simulink model "AssembledTEST1"  (R2016b)
settings: Solver=VariableStepAuto  StartTime=0.0  StopTime=60  RelTol=1e-9
values from neighbouring files (symbols this model uses):
  DOWN_0 = -xtrim(12)    [Comparison_NonLin.m]    (also in InitialiseJ31.m = 1830.0192; Trim.m)
  EAST_0 = xtrim(11)    [Comparison_NonLin.m]    (also in InitialiseJ31.m = 0; Trim.m)
  FLAP = 0    [InitialiseJ31.m]
  INERTIA = [IXX,IXY,IXZ;IXY,IYY,IYZ;IXZ,IYZ,IZZ]    [InitialiseJ31.m]
  NORTH_0 = xtrim(10)    [Comparison_NonLin.m]    (also in InitialiseJ31.m = 0; Trim.m)
  P_0 = xtrim(4)    [Comparison_NonLin.m]    (also in InitialiseJ31.m = 0; Trim.m)
  PHI_0 = xtrim(7)    [Comparison_NonLin.m]    (also in Trim.m)
  PSI_0 = xtrim(9)    [Comparison_NonLin.m]    (also in Trim.m)
  Q_0 = xtrim(5)    [Comparison_NonLin.m]    (also in InitialiseJ31.m = 0; Trim.m)
  R2D = 180/pi    (= 57.2957795131)    [InitialiseJ31.m]
  R_0 = xtrim(6)    [Comparison_NonLin.m]    (also in InitialiseJ31.m = 0; Trim.m)
  THETA_0 = xtrim(8)    [Comparison_NonLin.m]    (also in Trim.m)
  U_0 = xtrim(1)    [Comparison_NonLin.m]    (also in Trim.m)
  V_0 = xtrim(2)    [Comparison_NonLin.m]    (also in Trim.m)
  W_0 = xtrim(3)    [Comparison_NonLin.m]    (also in Trim.m)
undefined symbols (not defined in the file or in its folder): ail_data, Ap, Aw, b, beta0_data, c0, c_i, cdrag_data, CG, clean_wing_data, crt, CT_data, D, D0q_10, D0q_20, D0q_35, DCDi_data, DCM0b, Deh_f_on_data, Deh_on_data, df, Dqhq_data, e0, e_data10, e_data20, e_data35, elaw_0, elaw_1, elaw_2, flaps_lift_data, flaps_moment_data, flaps_tail_data, flaps_wing_data, fmc_data, fmf_data, fmn_data, fus_data, gamma_t, h_data10, h_data20, h_data35, it, iw, Iwn2, J_W, K1_data, k1f_data, k_data, L_r0_10f, L_r0_20f, L_r0_35f, l_t, ld_data, Lt, Lt_dash, Lv_b, Lv_h, Lv_n, mac, mach_ffr ... (+39)
libraries: aerolibasang x3, aerolibatmos2 x1
(part 3 of 5)

== system AssembledTEST1/Subsystem/Longitudinal Aerodynamics/Get Wing XZM/Get XZM ==
  D : Inport
  L : Inport  Port=2
  alpha : Inport  Port=3
  M0 : Inport  Port=4
  x : Inport  Port=5
  z : Inport  Port=6
  Add : Sum  Inputs=--
  Add1 : Sum  Inputs=+-
  Add2 : Sum  Inputs=-++
  Product{,1..5} (6 alike) : Product  RndMeth=Zero
  Trigonometric Function : Trigonometry
  Trigonometric Function1 : Trigonometry  Operator=cos
  X : Outport
  Z : Outport  Port=2
  M : Outport  Port=3
  wires:
  alpha/1 -> Trigonometric Function/1, Trigonometric Function1/1
  L/1 -> Product1/1, Product/1
  Trigonometric Function1/1 -> Product/2, Product2/1
  Trigonometric Function/1 -> Product1/2, Product3/1
  D/1 -> Product3/2, Product2/2
  Add/1 -> Product4/1, Z/1
  Product/1 -> Add/1
  Product3/1 -> Add/2
  Product1/1 -> Add1/1
  Product2/1 -> Add1/2
  Add1/1 -> Product5/1, X/1
  Product4/1 -> Add2/1
  Product5/1 -> Add2/2
  x/1 -> Product4/2
  Add2/1 -> M/1
  z/1 -> Product5/2
  M0/1 -> Add2/3

== system AssembledTEST1/Subsystem/Longitudinal Aerodynamics/Get Wing XZM/get_M0w ==
  Mach : Inport
  Flap : Inport  Port=2
  qbar : Inport  Port=3
  Add : Sum
  Add1 : Sum
  Constant2 : Constant
  Constant3 : Constant  Value=0
  Constant5 : Constant  Value=Sw
  Constant6 : Constant  Value=mac
  Multiport Switch : MultiPortSwitch  Inputs=4
  Product : Product  Inputs=4  RndMeth=Zero
  get_CM0W : Lookup  InputValues=clean_wing_data(:,1)  Table=clean_wing_data(:,7)
  get_delCM0a10 : Lookup  InputValues=flaps_moment_data(:,1)  Table=flaps_moment_data(:,2)
  get_delCM0a20 : Lookup  InputValues=flaps_moment_data(:,1)  Table=flaps_moment_data(:,3)
  get_delCM0a35 : Lookup  InputValues=flaps_moment_data(:,1)  Table=flaps_moment_data(:,4)
  M0 : Outport
  wires:
  Mach/1 -> get_delCM0a35/1, get_delCM0a20/1, get_delCM0a10/1, get_CM0W/1
  Constant2/1 -> Add/1
  Add/1 -> Multiport Switch/1
  Constant3/1 -> Multiport Switch/2
  get_delCM0a10/1 -> Multiport Switch/3
  get_delCM0a20/1 -> Multiport Switch/4
  get_delCM0a35/1 -> Multiport Switch/5
  Add1/1 -> Product/1
  Constant5/1 -> Product/2
  Constant6/1 -> Product/4
  Product/1 -> M0/1
  qbar/1 -> Product/3
  Flap/1 -> Add/2
  Multiport Switch/1 -> Add1/2
  get_CM0W/1 -> Add1/1

== system AssembledTEST1/Subsystem/Longitudinal Aerodynamics/get_CDvwbasic/get_DelCL0tw ==
  flap : Inport
  Mach : Inport  Port=2
  Add : Sum
  Constant1 : Constant
  Constant6 : Constant  Value=0
  Multiport Switch1 : MultiPortSwitch  Inputs=4
  get_DelCL0_10 : Lookup  InputValues=flaps_lift_data(:,1)  Table=flaps_lift_data(:,8)
  get_DelCL0_20 : Lookup  InputValues=flaps_lift_data(:,1)  Table=flaps_lift_data(:,9)
  get_DelCL0_35 : Lookup  InputValues=flaps_lift_data(:,1)  Table=flaps_lift_data(:,10)
  DelCL0tw : Outport
  wires:
  Constant6/1 -> Multiport Switch1/2
  get_DelCL0_10/1 -> Multiport Switch1/3
  get_DelCL0_20/1 -> Multiport Switch1/4
  get_DelCL0_35/1 -> Multiport Switch1/5
  Mach/1 -> get_DelCL0_10/1, get_DelCL0_20/1, get_DelCL0_35/1
  Multiport Switch1/1 -> DelCL0tw/1
  Add/1 -> Multiport Switch1/1
  flap/1 -> Add/1
  Constant1/1 -> Add/2

== system AssembledTEST1/Subsystem/Longitudinal Aerodynamics/get_CDvwbasic/get_kf ==
  flap : Inport
  Mach : Inport  Port=2
  Add : Sum
  Constant1 : Constant
  Constant6 : Constant  Value=0
  Multiport Switch1 : MultiPortSwitch  Inputs=4
  get_DelCL0_35 : Lookup  InputValues=flaps_lift_data(:,1)  Table=flaps_lift_data(:,13)
  get_kf_10 : Lookup  InputValues=flaps_lift_data(:,1)  Table=flaps_lift_data(:,11)
  get_kf_20 : Lookup  InputValues=flaps_lift_data(:,1)  Table=flaps_lift_data(:,12)
  kf : Outport
  wires:
  Constant6/1 -> Multiport Switch1/2
  get_kf_10/1 -> Multiport Switch1/3
  get_kf_20/1 -> Multiport Switch1/4
  get_DelCL0_35/1 -> Multiport Switch1/5
  Mach/1 -> get_kf_10/1, get_kf_20/1, get_DelCL0_35/1
  Multiport Switch1/1 -> kf/1
  Add/1 -> Multiport Switch1/1
  flap/1 -> Add/1
  Constant1/1 -> Add/2

== system AssembledTEST1/Subsystem/Powerplants and Slipstream/Subsystem2/Get_delDi ==
  In2 : Inport
  In1 : Inport  Port=2
  In3 : Inport  Port=3
  In4 : Inport  Port=4
  In5 : Inport  Port=5
  In6 : Inport  Port=6
  In7 : Inport  Port=7
  In8 : Inport  Port=8
  Constant1 : Constant  Value=Aw
  Constant2 : Constant  Value=Sw
  Constant3 : Constant  Value=b
  Constant4 : Constant  Value=D
  Get KDi : Lookup  InputValues=DCDi_data(:,1)  Table=DCDi_data(:,2)
  Get bar e/ep : Lookup  InputValues=DCDi_data(:,1)  Table=DCDi_data(:,3)
  GetDelCDi : MATLAB Function  TreatAsAtomicUnit=on
  Out1 : Outport
  wires:
  In2/1 -> Get KDi/1, Get bar e/ep/1
  Get KDi/1 -> GetDelCDi/1(KDi)
  Get bar e/ep/1 -> GetDelCDi/3(bar_e_ep)
  Constant2/1 -> GetDelCDi/9(Sw)
  Constant1/1 -> GetDelCDi/10(Aw)
  Constant3/1 -> GetDelCDi/11(b)
  Constant4/1 -> GetDelCDi/13(D)
  In1/1 -> GetDelCDi/2(alpha)
  In3/1 -> GetDelCDi/4(Xp)
  In4/1 -> GetDelCDi/5(Zp)
  In5/1 -> GetDelCDi/6(CLw)
  In6/1 -> GetDelCDi/7(deu_dap)
  GetDelCDi/1(delDi) -> Out1/1
  In7/1 -> GetDelCDi/8(qbar)
  In8/1 -> GetDelCDi/12(CDiw)

== system AssembledTEST1/Subsystem/Powerplants and Slipstream/Subsystem2/Get_delDi1 ==
  In2 : Inport
  In1 : Inport  Port=2
  In3 : Inport  Port=3
  In4 : Inport  Port=4
  In5 : Inport  Port=5
  In6 : Inport  Port=6
  In7 : Inport  Port=7
  In8 : Inport  Port=8
  Constant1 : Constant  Value=Aw
  Constant2 : Constant  Value=Sw
  Constant3 : Constant  Value=b
  Constant4 : Constant  Value=D
  Get KDi : Lookup  InputValues=DCDi_data(:,1)  Table=DCDi_data(:,2)
  Get bar e/ep : Lookup  InputValues=DCDi_data(:,1)  Table=DCDi_data(:,3)
  GetDelCDi : MATLAB Function  TreatAsAtomicUnit=on
  Out1 : Outport
  wires:
  In2/1 -> Get KDi/1, Get bar e/ep/1
  Get KDi/1 -> GetDelCDi/1(KDi)
  Get bar e/ep/1 -> GetDelCDi/3(bar_e_ep)
  Constant2/1 -> GetDelCDi/9(Sw)
  Constant1/1 -> GetDelCDi/10(Aw)
  Constant3/1 -> GetDelCDi/11(b)
  Constant4/1 -> GetDelCDi/13(D)
  In1/1 -> GetDelCDi/2(alpha)
  In3/1 -> GetDelCDi/4(Xp)
  In4/1 -> GetDelCDi/5(Zp)
  In5/1 -> GetDelCDi/6(CLw)
  In6/1 -> GetDelCDi/7(deu_dap)
  GetDelCDi/1(delDi) -> Out1/1
  In7/1 -> GetDelCDi/8(qbar)
  In8/1 -> GetDelCDi/12(CDiw)

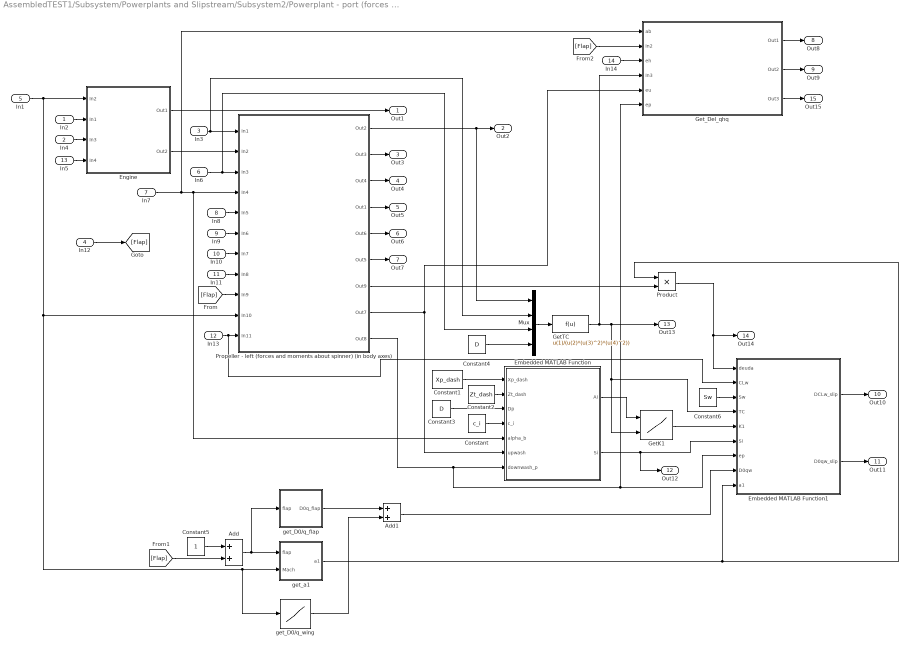
== system AssembledTEST1/Subsystem/Powerplants and Slipstream/Subsystem2/Powerplant - port (forces and moments about spinner) (in body axes) ==
  In2 : Inport
  In4 : Inport  Port=2
  In3 : Inport  Port=3
  In12 : Inport  Port=4
  In1 : Inport  Port=5
  In6 : Inport  Port=6
  In7 : Inport  Port=7
  In8 : Inport  Port=8
  In9 : Inport  Port=9
  In10 : Inport  Port=10
  In11 : Inport  Port=11
  In13 : Inport  Port=12
  In5 : Inport  Port=13
  In14 : Inport  Port=14
  Add : Sum
  Add1 : Sum
  Constant : Constant  Value=c_i
  Constant1 : Constant  Value=Xp_dash
  Constant2 : Constant  Value=Zt_dash
  Constant3 : Constant  Value=D
  Constant4 : Constant  Value=D
  Constant5 : Constant
  Constant6 : Constant  Value=Sw
  Embedded MATLAB Function : MATLAB Function  TreatAsAtomicUnit=on
  Embedded MATLAB Function1 : MATLAB Function  TreatAsAtomicUnit=on
  Engine : Subsystem
      mask Display:
      | port_label('output',1,'FFR [kg/h]')
      | port_label('output',2,'Power [SHP]')
      | port_label('input',1,'Mach')
      | port_label('input',2,'P_\infty [N/m^2]','texmode','on')
      | port_label('input',3,'T_\infty [K]','texmode','on')
      | port_label('input',4,'Throttle [%]')
  GetK1 : Lookup2D  RowIndex=Ai_ords  ColumnIndex=Tc_ords  Table=K1_data
  GetTC : Fcn  Expr=u(1)/(u(2)*(u(3)^2)*(u(4)^2))
  Get_Del_qhq : Subsystem
      mask Display:
      | port_label('output',1,'\Deltaq_h/q_\infty','texmode','on')
      | port_label('output',2,'(\Delta\epsilon_h)_{power}','texmode','on')
      | port_label('output',3,'\DeltaM_p/q_\infty','texmode','on')
      | port_label('input',1,'\alpha_b','texmode','on')
      | port_label('input',2,'Flap')
      | port_label('input',3,'(\epsilon_h)_{props off} [rad]','texmode','on')
      | port_label('input',4,'(S_W(T_c/prop))/(8R^2_p)','texmode','on')
      | port_label('input',5,'\epsilon_u [rad]','texmode','on')
      | port_label('input',6,'\epsilon_p [rad]','texmode','on')
  Mux : Mux
  Product : Product  RndMeth=Zero
  Propeller - left (forces and moments about spinner) (in body axes) : Subsystem
      mask Display:
      | port_label('output',1,'X [N]')
      | port_label('output',2,'Y [N]')
      | port_label('output',3,'Z [N]')
      | port_label('output',4,'L [Nm]')
      | port_label('output',5,'M [Nm]')
      | port_label('output',6,'N [Nm]')
      | port_label('output',8,'\epsilon_u [rad]','texmode','on')
      | port_label('output',9,'\epsilon_p [rad]','texmode','on')
      | port_label('output',7,'\delta\epsilon_u/\deltaC_L [rad]','texmode','on')
      | port_label('input',1,'\rho_\infty [kg/m^3]','texmode','on')
      | port_label('input',2,'Power [SHP]')
      | port_label('input',3,'V [m/s]')
      | port_label('input',4,'\alpha_b [rad]','texmode','on')
      | port_label('input',5,'\beta [rad]','texmode','on')
      | port_label('input',6,'p [rad/s]')
      | port_label('input',7,'q [rad/s]')
      | port_label('input',8,'r [rad/s]')
      | port_label('input',9,'Flap')
      | port_label('input',10,'Mach')
      | port_label('input',11,'C_{Lw}','texmode','on')
  get_D0/q_flap : Subsystem
  get_D0/q_wing : Lookup  InputValues=pdrag_data(:,1)  Table=pdrag_data(:,2)
  get_a1 : Subsystem
  Out1 : Outport
  Out2 : Outport  Port=2
  Out3 : Outport  Port=3
  Out4 : Outport  Port=4
  Out5 : Outport  Port=5
  Out6 : Outport  Port=6
  Out7 : Outport  Port=7
  Out8 : Outport  Port=8
  Out9 : Outport  Port=9
  Out10 : Outport  Port=10
  Out11 : Outport  Port=11
  Out12 : Outport  Port=12
  Out13 : Outport  Port=13
  Out14 : Outport  Port=14
  Out15 : Outport  Port=15
  wires:
  In1/1 -> Engine/1(In2), Propeller - left (forces and moments about spinner) (in body axes)/10(In10), get_a1/2(Mach), get_D0/q_wing/1
  Engine/2(Out2) -> Propeller - left (forces and moments about spinner) (in body axes)/2(In2)
  Engine/1(Out1) -> Out1/1
  In2/1 -> Engine/2(In1)
  In3/1 -> Propeller - left (forces and moments about spinner) (in body axes)/1(In1), Mux/2
  In4/1 -> Engine/3(In3)
  Propeller - left (forces and moments about spinner) (in body axes)/1(Out2) -> Out2/1, Mux/1
  In5/1 -> Engine/4(In4)
  In6/1 -> Propeller - left (forces and moments about spinner) (in body axes)/3(In3), Mux/3
  Propeller - left (forces and moments about spinner) (in body axes)/2(Out3) -> Out3/1
  In7/1 -> Propeller - left (forces and moments about spinner) (in body axes)/4(In4), Embedded MATLAB Function/5(alpha_b), Get_Del_qhq/1(ab)
  In8/1 -> Propeller - left (forces and moments about spinner) (in body axes)/5(In5)
  Propeller - left (forces and moments about spinner) (in body axes)/3(Out4) -> Out4/1
  In9/1 -> Propeller - left (forces and moments about spinner) (in body axes)/6(In6)
  In10/1 -> Propeller - left (forces and moments about spinner) (in body axes)/7(In7)
  Propeller - left (forces and moments about spinner) (in body axes)/4(Out1) -> Out5/1
  In11/1 -> Propeller - left (forces and moments about spinner) (in body axes)/8(In8)
  Propeller - left (forces and moments about spinner) (in body axes)/5(Out6) -> Out6/1
  Propeller - left (forces and moments about spinner) (in body axes)/6(Out5) -> Out7/1
  In13/1 -> Propeller - left (forces and moments about spinner) (in body axes)/11(In11), Embedded MATLAB Function1/2(CLw)
  Propeller - left (forces and moments about spinner) (in body axes)/8(Out7) -> Embedded MATLAB Function/6(upwash), Get_Del_qhq/5(eu)
  Propeller - left (forces and moments about spinner) (in body axes)/9(Out8) -> Embedded MATLAB Function/7(downwash_p), Get_Del_qhq/6(ep), Embedded MATLAB Function1/7(ep)
  Constant1/1 -> Embedded MATLAB Function/1(Xp_dash)
  Constant2/1 -> Embedded MATLAB Function/2(Zt_dash)
  Constant3/1 -> Embedded MATLAB Function/3(Dp)
  Constant/1 -> Embedded MATLAB Function/4(c_i)
  Embedded MATLAB Function/1(Ai) -> GetK1/1
  Mux/1 -> GetTC/1
  GetTC/1 -> GetK1/2, Embedded MATLAB Function1/4(TC), Out13/1, Get_Del_qhq/4(In3)
  Constant4/1 -> Mux/4
  Constant5/1 -> Add/1
  Add/1 -> get_a1/1(flap), get_D0/q_flap/1(flap)
  get_a1/1(a1) -> Product/1, Embedded MATLAB Function1/9(a1)
  Propeller - left (forces and moments about spinner) (in body axes)/7(Out9) -> Product/2
  Product/1 -> Out14/1, Embedded MATLAB Function1/1(deuda)
  Embedded MATLAB Function/2(Si) -> Out12/1, Embedded MATLAB Function1/6(Si)
  GetK1/1 -> Embedded MATLAB Function1/5(K1)
  Constant6/1 -> Embedded MATLAB Function1/3(Sw)
  get_D0/q_flap/1(D0q_flap) -> Add1/1
  get_D0/q_wing/1 -> Add1/2
  Add1/1 -> Embedded MATLAB Function1/8(D0qw)
  In12/1 -> [Flap]
  [Flap] -> Propeller - left (forces and moments about spinner) (in body axes)/9(In9)
  [Flap] -> Add/2
  [Flap] -> Get_Del_qhq/2(In2)
  In14/1 -> Get_Del_qhq/3(eh)
  Get_Del_qhq/1(Out1) -> Out8/1
  Embedded MATLAB Function1/1(DCLw_slip) -> Out10/1
  Embedded MATLAB Function1/2(D0qw_slip) -> Out11/1
  Get_Del_qhq/2(Out2) -> Out9/1
  Get_Del_qhq/3(Out3) -> Out15/1

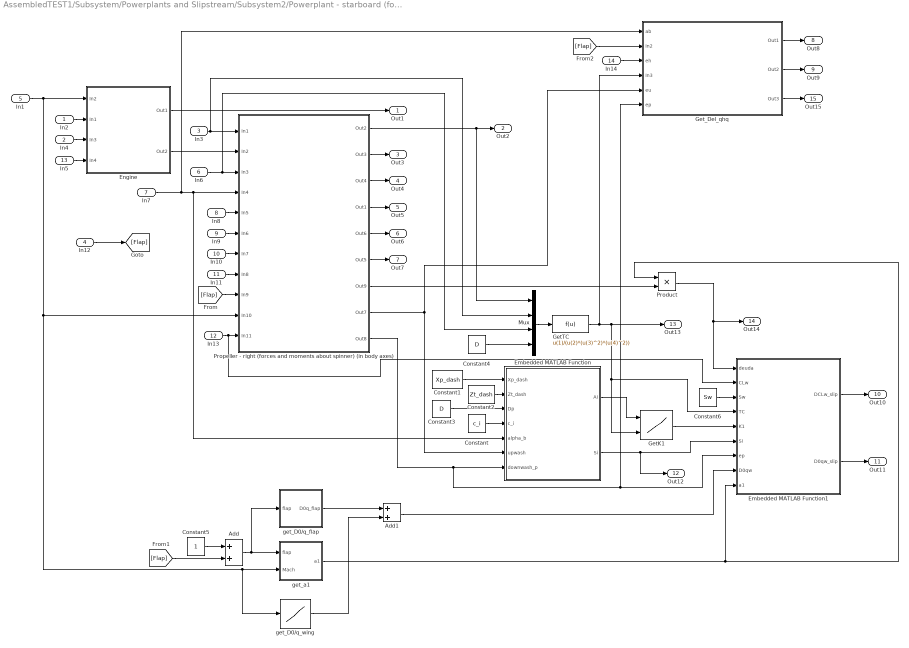
== system AssembledTEST1/Subsystem/Powerplants and Slipstream/Subsystem2/Powerplant - starboard (forces and moments about spinner) (in body axes) ==
  In2 : Inport
  In4 : Inport  Port=2
  In3 : Inport  Port=3
  In12 : Inport  Port=4
  In1 : Inport  Port=5
  In6 : Inport  Port=6
  In7 : Inport  Port=7
  In8 : Inport  Port=8
  In9 : Inport  Port=9
  In10 : Inport  Port=10
  In11 : Inport  Port=11
  In13 : Inport  Port=12
  In5 : Inport  Port=13
  In14 : Inport  Port=14
  Add : Sum
  Add1 : Sum
  Constant : Constant  Value=c_i
  Constant1 : Constant  Value=Xp_dash
  Constant2 : Constant  Value=Zt_dash
  Constant3 : Constant  Value=D
  Constant4 : Constant  Value=D
  Constant5 : Constant
  Constant6 : Constant  Value=Sw
  Embedded MATLAB Function : MATLAB Function  TreatAsAtomicUnit=on
  Embedded MATLAB Function1 : MATLAB Function  TreatAsAtomicUnit=on
  Engine : Subsystem
      mask Display:
      | port_label('output',1,'FFR [kg/h]')
      | port_label('output',2,'Power [SHP]')
      | port_label('input',1,'Mach')
      | port_label('input',2,'P_\infty [N/m^2]','texmode','on')
      | port_label('input',3,'T_\infty [K]','texmode','on')
      | port_label('input',4,'Throttle [%]')
  GetK1 : Lookup2D  RowIndex=Ai_ords  ColumnIndex=Tc_ords  Table=K1_data
  GetTC : Fcn  Expr=u(1)/(u(2)*(u(3)^2)*(u(4)^2))
  Get_Del_qhq : Subsystem
      mask Display:
      | port_label('output',1,'\Deltaq_h/q_\infty','texmode','on')
      | port_label('output',2,'(\Delta\epsilon_h)_{power}','texmode','on')
      | port_label('output',3,'\DeltaM_p/q_\infty','texmode','on')
      | port_label('input',1,'\alpha_b','texmode','on')
      | port_label('input',2,'Flap')
      | port_label('input',3,'(\epsilon_h)_{props off} [rad]','texmode','on')
      | port_label('input',4,'(S_W(T_c/prop))/(8R^2_p)','texmode','on')
      | port_label('input',5,'\epsilon_u [rad]','texmode','on')
      | port_label('input',6,'\epsilon_p [rad]','texmode','on')
  Mux : Mux
  Product : Product  RndMeth=Zero
  Propeller - right (forces and moments about spinner) (in body axes) : Subsystem
      mask Display:
      | port_label('output',1,'X [N]')
      | port_label('output',2,'Y [N]')
      | port_label('output',3,'Z [N]')
      | port_label('output',4,'L [Nm]')
      | port_label('output',5,'M [Nm]')
      | port_label('output',6,'N [Nm]')
      | port_label('output',8,'\epsilon_u [rad]','texmode','on')
      | port_label('output',9,'\epsilon_p [rad]','texmode','on')
      | port_label('output',7,'\delta\epsilon_u/\deltaC_L [rad]','texmode','on')
      | port_label('input',1,'\rho_\infty [kg/m^3]','texmode','on')
      | port_label('input',2,'Power [SHP]')
      | port_label('input',3,'V [m/s]')
      | port_label('input',4,'\alpha_b [rad]','texmode','on')
      | port_label('input',5,'\beta [rad]','texmode','on')
      | port_label('input',6,'p [rad/s]')
      | port_label('input',7,'q [rad/s]')
      | port_label('input',8,'r [rad/s]')
      | port_label('input',9,'Flap')
      | port_label('input',10,'Mach')
      | port_label('input',11,'C_{Lw}','texmode','on')
  get_D0/q_flap : Subsystem
  get_D0/q_wing : Lookup  InputValues=pdrag_data(:,1)  Table=pdrag_data(:,2)
  get_a1 : Subsystem
  Out1 : Outport
  Out2 : Outport  Port=2
  Out3 : Outport  Port=3
  Out4 : Outport  Port=4
  Out5 : Outport  Port=5
  Out6 : Outport  Port=6
  Out7 : Outport  Port=7
  Out8 : Outport  Port=8
  Out9 : Outport  Port=9
  Out10 : Outport  Port=10
  Out11 : Outport  Port=11
  Out12 : Outport  Port=12
  Out13 : Outport  Port=13
  Out14 : Outport  Port=14
  Out15 : Outport  Port=15
  wires:
  In1/1 -> Engine/1(In2), Propeller - right (forces and moments about spinner) (in body axes)/10(In10), get_a1/2(Mach), get_D0/q_wing/1
  Engine/2(Out2) -> Propeller - right (forces and moments about spinner) (in body axes)/2(In2)
  Engine/1(Out1) -> Out1/1
  In2/1 -> Engine/2(In1)
  In3/1 -> Propeller - right (forces and moments about spinner) (in body axes)/1(In1), Mux/2
  In4/1 -> Engine/3(In3)
  Propeller - right (forces and moments about spinner) (in body axes)/1(Out2) -> Out2/1, Mux/1
  In5/1 -> Engine/4(In4)
  In6/1 -> Propeller - right (forces and moments about spinner) (in body axes)/3(In3), Mux/3
  Propeller - right (forces and moments about spinner) (in body axes)/2(Out3) -> Out3/1
  In7/1 -> Propeller - right (forces and moments about spinner) (in body axes)/4(In4), Embedded MATLAB Function/5(alpha_b), Get_Del_qhq/1(ab)
  In8/1 -> Propeller - right (forces and moments about spinner) (in body axes)/5(In5)
  Propeller - right (forces and moments about spinner) (in body axes)/3(Out4) -> Out4/1
  In9/1 -> Propeller - right (forces and moments about spinner) (in body axes)/6(In6)
  In10/1 -> Propeller - right (forces and moments about spinner) (in body axes)/7(In7)
  Propeller - right (forces and moments about spinner) (in body axes)/4(Out1) -> Out5/1
  In11/1 -> Propeller - right (forces and moments about spinner) (in body axes)/8(In8)
  Propeller - right (forces and moments about spinner) (in body axes)/5(Out6) -> Out6/1
  Propeller - right (forces and moments about spinner) (in body axes)/6(Out5) -> Out7/1
  In13/1 -> Propeller - right (forces and moments about spinner) (in body axes)/11(In11), Embedded MATLAB Function1/2(CLw)
  Propeller - right (forces and moments about spinner) (in body axes)/8(Out7) -> Embedded MATLAB Function/6(upwash), Get_Del_qhq/5(eu)
  Propeller - right (forces and moments about spinner) (in body axes)/9(Out8) -> Embedded MATLAB Function/7(downwash_p), Get_Del_qhq/6(ep), Embedded MATLAB Function1/7(ep)
  Constant1/1 -> Embedded MATLAB Function/1(Xp_dash)
  Constant2/1 -> Embedded MATLAB Function/2(Zt_dash)
  Constant3/1 -> Embedded MATLAB Function/3(Dp)
  Constant/1 -> Embedded MATLAB Function/4(c_i)
  Embedded MATLAB Function/1(Ai) -> GetK1/1
  Mux/1 -> GetTC/1
  GetTC/1 -> Get_Del_qhq/4(In3), GetK1/2, Embedded MATLAB Function1/4(TC), Out13/1
  Constant4/1 -> Mux/4
  Constant5/1 -> Add/1
  Add/1 -> get_a1/1(flap), get_D0/q_flap/1(flap)
  get_a1/1(a1) -> Product/1, Embedded MATLAB Function1/9(a1)
  Propeller - right (forces and moments about spinner) (in body axes)/7(Out9) -> Product/2
  Product/1 -> Out14/1, Embedded MATLAB Function1/1(deuda)
  Embedded MATLAB Function/2(Si) -> Out12/1, Embedded MATLAB Function1/6(Si)
  GetK1/1 -> Embedded MATLAB Function1/5(K1)
  Constant6/1 -> Embedded MATLAB Function1/3(Sw)
  get_D0/q_flap/1(D0q_flap) -> Add1/1
  get_D0/q_wing/1 -> Add1/2
  Add1/1 -> Embedded MATLAB Function1/8(D0qw)
  In12/1 -> [Flap]
  [Flap] -> Propeller - right (forces and moments about spinner) (in body axes)/9(In9)
  [Flap] -> Add/2
  [Flap] -> Get_Del_qhq/2(In2)
  In14/1 -> Get_Del_qhq/3(eh)
  Get_Del_qhq/1(Out1) -> Out8/1
  Get_Del_qhq/2(Out2) -> Out9/1
  Embedded MATLAB Function1/1(DCLw_slip) -> Out10/1
  Embedded MATLAB Function1/2(D0qw_slip) -> Out11/1
  Get_Del_qhq/3(Out3) -> Out15/1

== system AssembledTEST1/Subsystem/Powerplants and Slipstream/Subsystem2/Subsystem ==
  In1 : Inport
  In2 : Inport  Port=2
  In5 : Inport  Port=3
  In3 : Inport  Port=4
  In4 : Inport  Port=5
  In6 : Inport  Port=6
  Add : Sum  Inputs=+-
  Add1 : Sum
  Constant : Constant
  Constant1 : Constant  Value=0.5
  Constant2 : Constant  Value=St
  Constant3 : Constant  Value=Sit
  Divide : Product  Inputs=*/***
  Product : Product  RndMeth=Zero
  Product1 : Product  RndMeth=Zero
  Product2 : Product  Inputs=4  RndMeth=Zero
  Out1 : Outport
  Out2 : Outport  Port=2
  wires:
  Product/1 -> Add/2
  Add/1 -> Product1/1
  Constant/1 -> Add1/2
  Add1/1 -> Product1/2
  Product1/1 -> Product2/1
  Constant1/1 -> Product2/2
  Constant2/1 -> Product2/3, Divide/2
  In1/1 -> Add/1
  In2/1 -> Product/1
  In3/1 -> Product/2
  Product2/1 -> Out1/1
  In4/1 -> Product2/4, Divide/1
  In5/1 -> Add1/1, Divide/4
  Divide/1 -> Out2/1
  Constant3/1 -> Divide/3
  In6/1 -> Divide/5

== system AssembledTEST1/Subsystem/Powerplants and Slipstream/Subsystem2/Subsystem1 ==
  In1 : Inport
  In2 : Inport  Port=2
  In5 : Inport  Port=3
  In3 : Inport  Port=4
  In4 : Inport  Port=5
  In6 : Inport  Port=6
  Add : Sum  Inputs=+-
  Add1 : Sum
  Constant : Constant
  Constant1 : Constant  Value=0.5
  Constant2 : Constant  Value=St
  Constant3 : Constant  Value=Sit
  Divide : Product  Inputs=*/***
  Product : Product  RndMeth=Zero
  Product1 : Product  RndMeth=Zero
  Product2 : Product  Inputs=4  RndMeth=Zero
  Out1 : Outport
  Out2 : Outport  Port=2
  wires:
  Product/1 -> Add/2
  Add/1 -> Product1/1
  Constant/1 -> Add1/2
  Add1/1 -> Product1/2
  Product1/1 -> Product2/1
  Constant1/1 -> Product2/2
  Constant2/1 -> Product2/3, Divide/2
  In1/1 -> Add/1
  In2/1 -> Product/1
  In3/1 -> Product/2
  Product2/1 -> Out1/1
  In4/1 -> Product2/4, Divide/1
  In5/1 -> Add1/1, Divide/4
  Divide/1 -> Out2/1
  Constant3/1 -> Divide/3
  In6/1 -> Divide/5

== system AssembledTEST1/Subsystem/Lateral//Directional Aerodynamics/getYLN/Subsystem/If Action Subsystem ==
  In1 : Inport
  Action Port : ActionPort  ActionType=else
  Out1 : Outport
  wires:
  In1/1 -> Out1/1

== system AssembledTEST1/Subsystem/Lateral//Directional Aerodynamics/getYLN/Subsystem/If Action Subsystem1 ==
  In1 : Inport
  Action Port : ActionPort  ActionType=then
  Out1 : Outport
  wires:
  In1/1 -> Out1/1

== system AssembledTEST1/Subsystem/Longitudinal Aerodynamics/Get Drag/get_CDvw/get_DelCL0tw ==
  flap : Inport
  Mach : Inport  Port=2
  Constant6 : Constant  Value=0
  Multiport Switch1 : MultiPortSwitch  Inputs=4
  get_DelCL0_10 : Lookup  InputValues=flaps_lift_data(:,1)  Table=flaps_lift_data(:,8)
  get_DelCL0_20 : Lookup  InputValues=flaps_lift_data(:,1)  Table=flaps_lift_data(:,9)
  get_DelCL0_35 : Lookup  InputValues=flaps_lift_data(:,1)  Table=flaps_lift_data(:,10)
  DelCL0tw : Outport
  wires:
  Constant6/1 -> Multiport Switch1/2
  get_DelCL0_10/1 -> Multiport Switch1/3
  get_DelCL0_20/1 -> Multiport Switch1/4
  get_DelCL0_35/1 -> Multiport Switch1/5
  flap/1 -> Multiport Switch1/1
  Mach/1 -> get_DelCL0_10/1, get_DelCL0_20/1, get_DelCL0_35/1
  Multiport Switch1/1 -> DelCL0tw/1

== system AssembledTEST1/Subsystem/Longitudinal Aerodynamics/Get Drag/get_CDvw/get_kf ==
  flap : Inport
  Mach : Inport  Port=2
  Constant6 : Constant  Value=0
  Multiport Switch1 : MultiPortSwitch  Inputs=4
  get_DelCL0_35 : Lookup  InputValues=flaps_lift_data(:,1)  Table=flaps_lift_data(:,13)
  get_kf_10 : Lookup  InputValues=flaps_lift_data(:,1)  Table=flaps_lift_data(:,11)
  get_kf_20 : Lookup  InputValues=flaps_lift_data(:,1)  Table=flaps_lift_data(:,12)
  kf : Outport
  wires:
  Constant6/1 -> Multiport Switch1/2
  get_kf_10/1 -> Multiport Switch1/3
  get_kf_20/1 -> Multiport Switch1/4
  get_DelCL0_35/1 -> Multiport Switch1/5
  flap/1 -> Multiport Switch1/1
  Mach/1 -> get_kf_10/1, get_kf_20/1, get_DelCL0_35/1
  Multiport Switch1/1 -> kf/1

== system AssembledTEST1/Subsystem/Longitudinal Aerodynamics/Get Wing & Tail Lift/get_tail_lift/get_e & de//da ==
  aoa_w : Inport
  alpha0 : Inport  Port=2
  Mach : Inport  Port=3
  Flap : Inport  Port=4
  Add : Sum
  Add1 : Sum
  Add2 : Sum  Inputs=-+
  Constant : Constant
  Constant1 : Constant  Value=e0
  Multiport Switch1 : MultiPortSwitch  Inputs=4
  Multiport Switch3 : MultiPortSwitch  Inputs=4
  Product : Product  RndMeth=Zero
  de/da-clean : Lookup  InputValues=tail_data(:,1)  Table=tail_data(:,2)
  de/da10 : Lookup  InputValues=flaps_tail_data(:,1)  Table=flaps_tail_data(:,2)
  de/da20 : Lookup  InputValues=flaps_tail_data(:,1)  Table=flaps_tail_data(:,3)
  de/da35 : Lookup  InputValues=flaps_tail_data(:,1)  Table=flaps_tail_data(:,4)
  e_10 : Lookup2D  RowIndex=M_ords  ColumnIndex=a  Table=e_data10
  e_20 : Lookup2D  RowIndex=M_ords  ColumnIndex=a  Table=e_data20
  e_35 : Lookup2D  RowIndex=M_ords  ColumnIndex=a  Table=e_data35
  e : Outport
  deda : Outport  Port=2
  wires:
  de/da-clean/1 -> Multiport Switch3/2
  de/da10/1 -> Multiport Switch3/3
  de/da20/1 -> Multiport Switch3/4
  de/da35/1 -> Multiport Switch3/5
  Mach/1 -> de/da-clean/1, de/da10/1, de/da20/1, de/da35/1, e_10/1, e_20/1, e_35/1
  Multiport Switch3/1 -> deda/1, Product/1
  Add/1 -> Multiport Switch3/1, Multiport Switch1/1
  Constant/1 -> Add/1
  Flap/1 -> Add/2
  Multiport Switch1/1 -> e/1
  Add1/1 -> Multiport Switch1/2
  Product/1 -> Add1/1
  Constant1/1 -> Add1/2
  e_10/1 -> Multiport Switch1/3
  alpha0/1 -> Add2/1
  aoa_w/1 -> Add2/2, e_10/2, e_20/2, e_35/2
  Add2/1 -> Product/2
  e_20/1 -> Multiport Switch1/4
  e_35/1 -> Multiport Switch1/5

== system AssembledTEST1/Subsystem/Longitudinal Aerodynamics/Get Wing & Tail Lift/get_wing_lift/If Action Subsystem ==
  In1 : Inport
  Action Port : ActionPort  ActionType=then
  CL : Outport
  wires:
  In1/1 -> CL/1

== system AssembledTEST1/Subsystem/Longitudinal Aerodynamics/Get Wing & Tail Lift/get_wing_lift/If Action Subsystem1 ==
  aoa_w : Inport
  alpha_star : Inport  Port=2
  CLmax : Inport  Port=3
  a1star : Inport  Port=4
  Action Port : ActionPort  ActionType=elseif
  Add : Sum  Inputs=+-
  Add1 : Sum  Inputs=+-
  Add2 : Sum  Inputs=+-
  Constant : Constant  Value=0.39
  Constant1 : Constant
  Constant2 : Constant  Value=0.3
  Divide : Product  Inputs=**/
  Fcn : Fcn  Expr=u(1)^1.3
  Product : Product  RndMeth=Zero
  CL : Outport
  wires:
  aoa_w/1 -> Add/1
  alpha_star/1 -> Add/2
  a1star/1 -> Divide/1
  Add/1 -> Divide/2
  Constant/1 -> Divide/3
  Constant1/1 -> Add1/1
  Divide/1 -> Add1/2
  Add1/1 -> Fcn/1
  Constant2/1 -> Product/1
  Fcn/1 -> Product/2
  CLmax/1 -> Add2/1
  Product/1 -> Add2/2
  Add2/1 -> CL/1

== system AssembledTEST1/Subsystem/Longitudinal Aerodynamics/Get Wing & Tail Lift/get_wing_lift/If Action Subsystem2 ==
  a1 : Inport
  alpha_0 : Inport  Port=2
  n : Inport  Port=3
  aoa_w : Inport  Port=4
  Action Port : ActionPort  ActionType=else
  Add : Sum  Inputs=+-
  Fcn : Fcn  Expr=(cos(u(1)))^(u(2))
  Mux : Mux  Inputs=2
  Product : Product  Inputs=3  RndMeth=Zero
  CL : Outport
  wires:
  aoa_w/1 -> Add/1
  alpha_0/1 -> Add/2
  Add/1 -> Mux/1, Product/2
  n/1 -> Mux/2
  Mux/1 -> Fcn/1
  a1/1 -> Product/1
  Fcn/1 -> Product/3
  Product/1 -> CL/1

== system AssembledTEST1/Subsystem/Longitudinal Aerodynamics/Get Wing & Tail Lift/get_wing_lift/get_CLmax ==
  flap : Inport
  Mach : Inport  Port=2
  CLmax_clean : Lookup  InputValues=clean_wing_data(:,1)  Table=clean_wing_data(:,6)
  CLmax_flaps10 : Lookup  InputValues=flaps_wing_data(:,1)  Table=flaps_wing_data(:,14)
  CLmax_flaps20 : Lookup  InputValues=flaps_wing_data(:,1)  Table=flaps_wing_data(:,17)
  CLmax_flaps35 : Lookup  InputValues=flaps_wing_data(:,1)  Table=flaps_wing_data(:,20)
  Multiport Switch : MultiPortSwitch  Inputs=4
  CLmax : Outport
  wires:
  Mach/1 -> CLmax_flaps35/1, CLmax_flaps20/1, CLmax_flaps10/1, CLmax_clean/1
  CLmax_clean/1 -> Multiport Switch/2
  CLmax_flaps10/1 -> Multiport Switch/3
  CLmax_flaps20/1 -> Multiport Switch/4
  CLmax_flaps35/1 -> Multiport Switch/5
  flap/1 -> Multiport Switch/1
  Multiport Switch/1 -> CLmax/1

== system AssembledTEST1/Subsystem/Longitudinal Aerodynamics/Get Wing & Tail Lift/get_wing_lift/get_a1 ==
  flap : Inport
  Mach : Inport  Port=2
  Multiport Switch : MultiPortSwitch  Inputs=4
  a1_clean : Lookup  InputValues=clean_wing_data(:,1)  Table=clean_wing_data(:,2)
  a1_flaps10 : Lookup  InputValues=flaps_wing_data(:,1)  Table=flaps_wing_data(:,3)
  a1_flaps20 : Lookup  InputValues=flaps_wing_data(:,1)  Table=flaps_wing_data(:,6)
  a1_flaps35 : Lookup  InputValues=flaps_wing_data(:,1)  Table=flaps_wing_data(:,9)
  a1 : Outport
  wires:
  Mach/1 -> a1_flaps35/1, a1_flaps20/1, a1_flaps10/1, a1_clean/1
  a1_clean/1 -> Multiport Switch/2
  a1_flaps10/1 -> Multiport Switch/3
  a1_flaps20/1 -> Multiport Switch/4
  a1_flaps35/1 -> Multiport Switch/5
  flap/1 -> Multiport Switch/1
  Multiport Switch/1 -> a1/1

== system AssembledTEST1/Subsystem/Longitudinal Aerodynamics/Get Wing & Tail Lift/get_wing_lift/get_a1star ==
  flap : Inport
  Mach : Inport  Port=2
  Multiport Switch : MultiPortSwitch  Inputs=4
  a1star_clean : Lookup  InputValues=clean_wing_data(:,1)  Table=clean_wing_data(:,2)
  a1star_flaps10 : Lookup  InputValues=flaps_wing_data(:,1)  Table=flaps_wing_data(:,12)
  a1star_flaps20 : Lookup  InputValues=flaps_wing_data(:,1)  Table=flaps_wing_data(:,15)
  a1star_flaps35 : Lookup  InputValues=flaps_wing_data(:,1)  Table=flaps_wing_data(:,18)
  a1star : Outport
  wires:
  Mach/1 -> a1star_flaps35/1, a1star_flaps20/1, a1star_flaps10/1, a1star_clean/1
  a1star_clean/1 -> Multiport Switch/2
  a1star_flaps10/1 -> Multiport Switch/3
  a1star_flaps20/1 -> Multiport Switch/4
  a1star_flaps35/1 -> Multiport Switch/5
  flap/1 -> Multiport Switch/1
  Multiport Switch/1 -> a1star/1

== system AssembledTEST1/Subsystem/Longitudinal Aerodynamics/Get Wing & Tail Lift/get_wing_lift/get_alpha0 ==
  flap : Inport
  Mach : Inport  Port=2
  Multiport Switch : MultiPortSwitch  Inputs=4
  alpha0_clean : Lookup  InputValues=clean_wing_data(:,1)  Table=clean_wing_data(:,3)
  alpha0_flaps10 : Lookup  InputValues=flaps_wing_data(:,1)  Table=flaps_wing_data(:,4)
  alpha0_flaps20 : Lookup  InputValues=flaps_wing_data(:,1)  Table=flaps_wing_data(:,7)
  alpha0_flaps35 : Lookup  InputValues=flaps_wing_data(:,1)  Table=flaps_wing_data(:,10)
  alpha0 : Outport
  wires:
  Mach/1 -> alpha0_flaps35/1, alpha0_flaps20/1, alpha0_flaps10/1, alpha0_clean/1
  alpha0_clean/1 -> Multiport Switch/2
  alpha0_flaps10/1 -> Multiport Switch/3
  alpha0_flaps20/1 -> Multiport Switch/4
  alpha0_flaps35/1 -> Multiport Switch/5
  flap/1 -> Multiport Switch/1
  Multiport Switch/1 -> alpha0/1

== system AssembledTEST1/Subsystem/Longitudinal Aerodynamics/Get Wing & Tail Lift/get_wing_lift/get_alpha_star ==
  flap : Inport
  Mach : Inport  Port=2
  Multiport Switch : MultiPortSwitch  Inputs=4
  alpha_star_clean : Lookup  InputValues=clean_wing_data(:,1)  Table=clean_wing_data(:,4)
  alpha_star_flaps10 : Lookup  InputValues=flaps_wing_data(:,1)  Table=flaps_wing_data(:,5)
  alpha_star_flaps20 : Lookup  InputValues=flaps_wing_data(:,1)  Table=flaps_wing_data(:,8)
  alpha_star_flaps35 : Lookup  InputValues=flaps_wing_data(:,1)  Table=flaps_wing_data(:,11)
  alpha_star : Outport
  wires:
  Mach/1 -> alpha_star_flaps35/1, alpha_star_flaps20/1, alpha_star_flaps10/1, alpha_star_clean/1
  alpha_star_clean/1 -> Multiport Switch/2
  alpha_star_flaps10/1 -> Multiport Switch/3
  alpha_star_flaps20/1 -> Multiport Switch/4
  alpha_star_flaps35/1 -> Multiport Switch/5
  flap/1 -> Multiport Switch/1
  Multiport Switch/1 -> alpha_star/1

== system AssembledTEST1/Subsystem/Longitudinal Aerodynamics/Get Wing & Tail Lift/get_wing_lift/get_aoa_max ==
  flap : Inport
  Mach : Inport  Port=2
  Multiport Switch : MultiPortSwitch  Inputs=4
  aoa_max_clean : Lookup  InputValues=clean_wing_data(:,1)  Table=clean_wing_data(:,5)
  aoa_max_flaps10 : Lookup  InputValues=flaps_wing_data(:,1)  Table=flaps_wing_data(:,13)
  aoa_max_flaps20 : Lookup  InputValues=flaps_wing_data(:,1)  Table=flaps_wing_data(:,16)
  aoa_max_flaps35 : Lookup  InputValues=flaps_wing_data(:,1)  Table=flaps_wing_data(:,19)
  aoa_max : Outport
  wires:
  Mach/1 -> aoa_max_flaps35/1, aoa_max_flaps20/1, aoa_max_flaps10/1, aoa_max_clean/1
  aoa_max_clean/1 -> Multiport Switch/2
  aoa_max_flaps10/1 -> Multiport Switch/3
  aoa_max_flaps20/1 -> Multiport Switch/4
  aoa_max_flaps35/1 -> Multiport Switch/5
  flap/1 -> Multiport Switch/1
  Multiport Switch/1 -> aoa_max/1

== system AssembledTEST1/Subsystem/Longitudinal Aerodynamics/Get Wing & Tail Lift/get_wing_lift/get_aoa_w ==
  aoa : Inport
  V : Inport  Port=2
  xcg : Inport  Port=3
  q : Inport  Port=4
  delh : Inport  Port=5
  Add{1..4} (4 alike) : Sum
  Add5 : Sum  Inputs=+-+
  Constant1 : Constant  Value=xb0
  Constant2 : Constant  Value=c0
  Constant3 : Constant  Value=iw
  Divide3 : Product  Inputs=/*
  Fcn : Fcn  Expr=cos(u(1))
  Fcn1 : Fcn  Expr=sin(u(1))
  Fcn2 : Fcn  Expr=atan(u(1))
  Fcn3 : Fcn  Expr=u(1)*u(1)
  Fcn4 : Fcn  Expr=u(1)*u(1)
  Fcn5 : Fcn  Expr=sqrt(u(1))
  Gain : Gain  Gain=0.3
  Gain1 : Gain  Gain=-1
  Product : Product  RndMeth=Zero
  Product1 : Product  RndMeth=Zero
  Product2 : Product  RndMeth=Zero
  aoa_w : Outport
  Vw : Outport  Port=2
  xac_w : Outport  Port=3
  wires:
  Constant2/1 -> Gain/1
  Add1/1 -> Product/2
  aoa/1 -> Fcn/1, Fcn1/1
  Fcn1/1 -> Product2/1
  V/1 -> Product1/1, Product2/2
  Fcn/1 -> Product1/2
  Product2/1 -> Add2/1
  Product/1 -> Add2/2
  Product1/1 -> Divide3/1, Fcn4/1
  Add2/1 -> Divide3/2, Fcn3/1
  Divide3/1 -> Fcn2/1
  xcg/1 -> Add1/1
  q/1 -> Product/1
  Constant3/1 -> Add3/1
  Fcn2/1 -> Add3/2
  Add3/1 -> aoa_w/1
  Fcn4/1 -> Add4/1
  Fcn3/1 -> Add4/2
  Add4/1 -> Fcn5/1
  Fcn5/1 -> Vw/1
  Add5/1 -> Add1/2, Gain1/1
  Constant1/1 -> Add5/1
  Gain/1 -> Add5/2
  Gain1/1 -> xac_w/1
  delh/1 -> Add5/3

== system AssembledTEST1/Subsystem/Longitudinal Aerodynamics/Get Wing & Tail Lift/get_wing_lift/get_delh ==
  flap : Inport
  aoa : Inport  Port=2
  Mach : Inport  Port=3
  Add : Sum
  Constant3 : Constant  Value=0
  Gain : Gain  Gain=mac
  Gain1 : Gain  Gain=c0
  Multiport Switch : MultiPortSwitch  Inputs=4
  get_delxh : Lookup  InputValues=clean_wing_data(:,1)  Table=clean_wing_data(:,8)
  h_10 : Lookup2D  RowIndex=a_h  ColumnIndex=M_ords  Table=h_data10
  h_20 : Lookup2D  RowIndex=a_h  ColumnIndex=M_ords  Table=h_data20
  h_35 : Lookup2D  RowIndex=a_h  ColumnIndex=M_ords  Table=h_data35
  delh : Outport
  wires:
  Constant3/1 -> Multiport Switch/2
  h_10/1 -> Multiport Switch/3
  h_20/1 -> Multiport Switch/4
  h_35/1 -> Multiport Switch/5
  flap/1 -> Multiport Switch/1
  aoa/1 -> h_10/1, h_20/1, h_35/1
  Mach/1 -> h_10/2, h_20/2, h_35/2, get_delxh/1
  Add/1 -> delh/1
  Multiport Switch/1 -> Gain/1
  Gain/1 -> Add/1
  get_delxh/1 -> Gain1/1
  Gain1/1 -> Add/2

== system AssembledTEST1/Subsystem/Longitudinal Aerodynamics/Get Wing & Tail Lift/get_wing_lift/get_n ==
  flap : Inport
  Mach : Inport  Port=2
  Constant2 : Constant  Value=0
  Lookup Table1 : Lookup  InputValues=flaps_wing_data(:,1)  Table=flaps_wing_data(:,2)
  Lookup Table2 : Lookup  InputValues=flaps_wing_data(:,1)  Table=flaps_wing_data(:,2)
  Lookup Table3 : Lookup  InputValues=flaps_wing_data(:,1)  Table=flaps_wing_data(:,2)
  Multiport Switch1 : MultiPortSwitch  Inputs=4
  n : Outport
  wires:
  Lookup Table3/1 -> Multiport Switch1/5
  Lookup Table2/1 -> Multiport Switch1/4
  Constant2/1 -> Multiport Switch1/2
  Lookup Table1/1 -> Multiport Switch1/3
  flap/1 -> Multiport Switch1/1
  Mach/1 -> Lookup Table1/1, Lookup Table2/1, Lookup Table3/1
  Multiport Switch1/1 -> n/1

== system AssembledTEST1/Subsystem/Longitudinal Aerodynamics/Get Wing & Tail Lift/get_wing_lift_basic/If Action Subsystem ==
  In1 : Inport
  Action Port : ActionPort  ActionType=then
  CL : Outport
  wires:
  In1/1 -> CL/1

== system AssembledTEST1/Subsystem/Longitudinal Aerodynamics/Get Wing & Tail Lift/get_wing_lift_basic/If Action Subsystem1 ==
  aoa_w : Inport
  alpha_star : Inport  Port=2
  CLmax : Inport  Port=3
  a1star : Inport  Port=4
  Action Port : ActionPort  ActionType=elseif
  Add : Sum  Inputs=+-
  Add1 : Sum  Inputs=+-
  Add2 : Sum  Inputs=+-
  Constant : Constant  Value=0.39
  Constant1 : Constant
  Constant2 : Constant  Value=0.3
  Divide : Product  Inputs=**/
  Fcn : Fcn  Expr=u(1)^1.3
  Product : Product  RndMeth=Zero
  CL : Outport
  wires:
  aoa_w/1 -> Add/1
  alpha_star/1 -> Add/2
  a1star/1 -> Divide/1
  Add/1 -> Divide/2
  Constant/1 -> Divide/3
  Constant1/1 -> Add1/1
  Divide/1 -> Add1/2
  Add1/1 -> Fcn/1
  Constant2/1 -> Product/1
  Fcn/1 -> Product/2
  CLmax/1 -> Add2/1
  Product/1 -> Add2/2
  Add2/1 -> CL/1

== system AssembledTEST1/Subsystem/Longitudinal Aerodynamics/Get Wing & Tail Lift/get_wing_lift_basic/If Action Subsystem2 ==
  a1 : Inport
  alpha_0 : Inport  Port=2
  n : Inport  Port=3
  aoa_w : Inport  Port=4
  Action Port : ActionPort  ActionType=else
  Add : Sum  Inputs=+-
  Fcn : Fcn  Expr=(cos(u(1)))^(u(2))
  Mux : Mux  Inputs=2
  Product : Product  Inputs=3  RndMeth=Zero
  CL : Outport
  wires:
  aoa_w/1 -> Add/1
  alpha_0/1 -> Add/2
  Add/1 -> Mux/1, Product/2
  n/1 -> Mux/2
  Mux/1 -> Fcn/1
  a1/1 -> Product/1
  Fcn/1 -> Product/3
  Product/1 -> CL/1

== system AssembledTEST1/Subsystem/Longitudinal Aerodynamics/Get Wing & Tail Lift/get_wing_lift_basic/get_CLmax ==
  flap : Inport
  Mach : Inport  Port=2
  CLmax_clean : Lookup  InputValues=clean_wing_data(:,1)  Table=clean_wing_data(:,6)
  CLmax_flaps10 : Lookup  InputValues=flaps_wing_data(:,1)  Table=flaps_wing_data(:,14)
  CLmax_flaps20 : Lookup  InputValues=flaps_wing_data(:,1)  Table=flaps_wing_data(:,17)
  CLmax_flaps35 : Lookup  InputValues=flaps_wing_data(:,1)  Table=flaps_wing_data(:,20)
  Multiport Switch : MultiPortSwitch  Inputs=4
  CLmax : Outport
  wires:
  Mach/1 -> CLmax_flaps35/1, CLmax_flaps20/1, CLmax_flaps10/1, CLmax_clean/1
  CLmax_clean/1 -> Multiport Switch/2
  CLmax_flaps10/1 -> Multiport Switch/3
  CLmax_flaps20/1 -> Multiport Switch/4
  CLmax_flaps35/1 -> Multiport Switch/5
  flap/1 -> Multiport Switch/1
  Multiport Switch/1 -> CLmax/1

== system AssembledTEST1/Subsystem/Longitudinal Aerodynamics/Get Wing & Tail Lift/get_wing_lift_basic/get_a1 ==
  flap : Inport
  Mach : Inport  Port=2
  Multiport Switch : MultiPortSwitch  Inputs=4
  a1_clean : Lookup  InputValues=clean_wing_data(:,1)  Table=clean_wing_data(:,2)
  a1_flaps10 : Lookup  InputValues=flaps_wing_data(:,1)  Table=flaps_wing_data(:,3)
  a1_flaps20 : Lookup  InputValues=flaps_wing_data(:,1)  Table=flaps_wing_data(:,6)
  a1_flaps35 : Lookup  InputValues=flaps_wing_data(:,1)  Table=flaps_wing_data(:,9)
  a1 : Outport
  wires:
  Mach/1 -> a1_flaps35/1, a1_flaps20/1, a1_flaps10/1, a1_clean/1
  a1_clean/1 -> Multiport Switch/2
  a1_flaps10/1 -> Multiport Switch/3
  a1_flaps20/1 -> Multiport Switch/4
  a1_flaps35/1 -> Multiport Switch/5
  flap/1 -> Multiport Switch/1
  Multiport Switch/1 -> a1/1

== system AssembledTEST1/Subsystem/Longitudinal Aerodynamics/Get Wing & Tail Lift/get_wing_lift_basic/get_a1star ==
  flap : Inport
  Mach : Inport  Port=2
  Multiport Switch : MultiPortSwitch  Inputs=4
  a1star_clean : Lookup  InputValues=clean_wing_data(:,1)  Table=clean_wing_data(:,2)
  a1star_flaps10 : Lookup  InputValues=flaps_wing_data(:,1)  Table=flaps_wing_data(:,12)
  a1star_flaps20 : Lookup  InputValues=flaps_wing_data(:,1)  Table=flaps_wing_data(:,15)
  a1star_flaps35 : Lookup  InputValues=flaps_wing_data(:,1)  Table=flaps_wing_data(:,18)
  a1star : Outport
  wires:
  Mach/1 -> a1star_flaps35/1, a1star_flaps20/1, a1star_flaps10/1, a1star_clean/1
  a1star_clean/1 -> Multiport Switch/2
  a1star_flaps10/1 -> Multiport Switch/3
  a1star_flaps20/1 -> Multiport Switch/4
  a1star_flaps35/1 -> Multiport Switch/5
  flap/1 -> Multiport Switch/1
  Multiport Switch/1 -> a1star/1

== system AssembledTEST1/Subsystem/Longitudinal Aerodynamics/Get Wing & Tail Lift/get_wing_lift_basic/get_alpha0 ==
  flap : Inport
  Mach : Inport  Port=2
  Multiport Switch : MultiPortSwitch  Inputs=4
  alpha0_clean : Lookup  InputValues=clean_wing_data(:,1)  Table=clean_wing_data(:,3)
  alpha0_flaps10 : Lookup  InputValues=flaps_wing_data(:,1)  Table=flaps_wing_data(:,4)
  alpha0_flaps20 : Lookup  InputValues=flaps_wing_data(:,1)  Table=flaps_wing_data(:,7)
  alpha0_flaps35 : Lookup  InputValues=flaps_wing_data(:,1)  Table=flaps_wing_data(:,10)
  alpha0 : Outport
  wires:
  Mach/1 -> alpha0_flaps35/1, alpha0_flaps20/1, alpha0_flaps10/1, alpha0_clean/1
  alpha0_clean/1 -> Multiport Switch/2
  alpha0_flaps10/1 -> Multiport Switch/3
  alpha0_flaps20/1 -> Multiport Switch/4
  alpha0_flaps35/1 -> Multiport Switch/5
  flap/1 -> Multiport Switch/1
  Multiport Switch/1 -> alpha0/1

== system AssembledTEST1/Subsystem/Longitudinal Aerodynamics/Get Wing & Tail Lift/get_wing_lift_basic/get_alpha_star ==
  flap : Inport
  Mach : Inport  Port=2
  Multiport Switch : MultiPortSwitch  Inputs=4
  alpha_star_clean : Lookup  InputValues=clean_wing_data(:,1)  Table=clean_wing_data(:,4)
  alpha_star_flaps10 : Lookup  InputValues=flaps_wing_data(:,1)  Table=flaps_wing_data(:,5)
  alpha_star_flaps20 : Lookup  InputValues=flaps_wing_data(:,1)  Table=flaps_wing_data(:,8)
  alpha_star_flaps35 : Lookup  InputValues=flaps_wing_data(:,1)  Table=flaps_wing_data(:,11)
  alpha_star : Outport
  wires:
  Mach/1 -> alpha_star_flaps35/1, alpha_star_flaps20/1, alpha_star_flaps10/1, alpha_star_clean/1
  alpha_star_clean/1 -> Multiport Switch/2
  alpha_star_flaps10/1 -> Multiport Switch/3
  alpha_star_flaps20/1 -> Multiport Switch/4
  alpha_star_flaps35/1 -> Multiport Switch/5
  flap/1 -> Multiport Switch/1
  Multiport Switch/1 -> alpha_star/1

== system AssembledTEST1/Subsystem/Longitudinal Aerodynamics/Get Wing & Tail Lift/get_wing_lift_basic/get_aoa_max ==
  flap : Inport
  Mach : Inport  Port=2
  Multiport Switch : MultiPortSwitch  Inputs=4
  aoa_max_clean : Lookup  InputValues=clean_wing_data(:,1)  Table=clean_wing_data(:,5)
  aoa_max_flaps10 : Lookup  InputValues=flaps_wing_data(:,1)  Table=flaps_wing_data(:,13)
  aoa_max_flaps20 : Lookup  InputValues=flaps_wing_data(:,1)  Table=flaps_wing_data(:,16)
  aoa_max_flaps35 : Lookup  InputValues=flaps_wing_data(:,1)  Table=flaps_wing_data(:,19)
  aoa_max : Outport
  wires:
  Mach/1 -> aoa_max_flaps35/1, aoa_max_flaps20/1, aoa_max_flaps10/1, aoa_max_clean/1
  aoa_max_clean/1 -> Multiport Switch/2
  aoa_max_flaps10/1 -> Multiport Switch/3
  aoa_max_flaps20/1 -> Multiport Switch/4
  aoa_max_flaps35/1 -> Multiport Switch/5
  flap/1 -> Multiport Switch/1
  Multiport Switch/1 -> aoa_max/1

== system AssembledTEST1/Subsystem/Longitudinal Aerodynamics/Get Wing & Tail Lift/get_wing_lift_basic/get_aoa_w ==
  aoa : Inport
  V : Inport  Port=2
  xcg : Inport  Port=3
  q : Inport  Port=4
  delh : Inport  Port=5
  Add{1..4} (4 alike) : Sum
  Add5 : Sum  Inputs=+-+
  Constant1 : Constant  Value=xb0
  Constant2 : Constant  Value=c0
  Constant3 : Constant  Value=iw
  Divide3 : Product  Inputs=/*
  Fcn : Fcn  Expr=cos(u(1))
  Fcn1 : Fcn  Expr=sin(u(1))
  Fcn2 : Fcn  Expr=atan(u(1))
  Fcn3 : Fcn  Expr=u(1)*u(1)
  Fcn4 : Fcn  Expr=u(1)*u(1)
  Fcn5 : Fcn  Expr=sqrt(u(1))
  Gain : Gain  Gain=0.3
  Gain1 : Gain  Gain=-1
  Product : Product  RndMeth=Zero
  Product1 : Product  RndMeth=Zero
  Product2 : Product  RndMeth=Zero
  aoa_w : Outport
  Vw : Outport  Port=2
  xac_w : Outport  Port=3
  wires:
  Constant2/1 -> Gain/1
  Add1/1 -> Product/2
  aoa/1 -> Fcn/1, Fcn1/1
  Fcn1/1 -> Product2/1
  V/1 -> Product1/1, Product2/2
  Fcn/1 -> Product1/2
  Product2/1 -> Add2/1
  Product/1 -> Add2/2
  Product1/1 -> Divide3/1, Fcn4/1
  Add2/1 -> Divide3/2, Fcn3/1
  Divide3/1 -> Fcn2/1
  xcg/1 -> Add1/1
  q/1 -> Product/1
  Constant3/1 -> Add3/1
  Fcn2/1 -> Add3/2
  Add3/1 -> aoa_w/1
  Fcn4/1 -> Add4/1
  Fcn3/1 -> Add4/2
  Add4/1 -> Fcn5/1
  Fcn5/1 -> Vw/1
  Add5/1 -> Add1/2, Gain1/1
  Constant1/1 -> Add5/1
  Gain/1 -> Add5/2
  Gain1/1 -> xac_w/1
  delh/1 -> Add5/3

== system AssembledTEST1/Subsystem/Longitudinal Aerodynamics/Get Wing & Tail Lift/get_wing_lift_basic/get_delh ==
  flap : Inport
  aoa : Inport  Port=2
  Mach : Inport  Port=3
  Add : Sum
  Constant3 : Constant  Value=0
  Gain : Gain  Gain=mac
  Gain1 : Gain  Gain=c0
  Multiport Switch : MultiPortSwitch  Inputs=4
  get_delxh : Lookup  InputValues=clean_wing_data(:,1)  Table=clean_wing_data(:,8)
  h_10 : Lookup2D  RowIndex=a_h  ColumnIndex=M_ords  Table=h_data10
  h_20 : Lookup2D  RowIndex=a_h  ColumnIndex=M_ords  Table=h_data20
  h_35 : Lookup2D  RowIndex=a_h  ColumnIndex=M_ords  Table=h_data35
  delh : Outport
  wires:
  Constant3/1 -> Multiport Switch/2
  h_10/1 -> Multiport Switch/3
  h_20/1 -> Multiport Switch/4
  h_35/1 -> Multiport Switch/5
  flap/1 -> Multiport Switch/1
  aoa/1 -> h_10/1, h_20/1, h_35/1
  Mach/1 -> h_10/2, h_20/2, h_35/2, get_delxh/1
  Add/1 -> delh/1
  Multiport Switch/1 -> Gain/1
  Gain/1 -> Add/1
  get_delxh/1 -> Gain1/1
  Gain1/1 -> Add/2

== system AssembledTEST1/Subsystem/Longitudinal Aerodynamics/Get Wing & Tail Lift/get_wing_lift_basic/get_n ==
  flap : Inport
  Mach : Inport  Port=2
  Constant2 : Constant  Value=0
  Lookup Table1 : Lookup  InputValues=flaps_wing_data(:,1)  Table=flaps_wing_data(:,2)
  Lookup Table2 : Lookup  InputValues=flaps_wing_data(:,1)  Table=flaps_wing_data(:,2)
  Lookup Table3 : Lookup  InputValues=flaps_wing_data(:,1)  Table=flaps_wing_data(:,2)
  Multiport Switch1 : MultiPortSwitch  Inputs=4
  n : Outport
  wires:
  Lookup Table3/1 -> Multiport Switch1/5
  Lookup Table2/1 -> Multiport Switch1/4
  Constant2/1 -> Multiport Switch1/2
  Lookup Table1/1 -> Multiport Switch1/3
  flap/1 -> Multiport Switch1/1
  Mach/1 -> Lookup Table1/1, Lookup Table2/1, Lookup Table3/1
  Multiport Switch1/1 -> n/1

== system AssembledTEST1/Subsystem/Powerplants and Slipstream/Subsystem2/Powerplant - port (forces and moments about spinner) (in body axes)/Engine ==
  In2 : Inport
  In1 : Inport  Port=2
  In3 : Inport  Port=3
  In4 : Inport  Port=4
  % throttle to FFR : Gain  Gain=2.5
  Altitude effect on FFR : Fcn  Expr=u(3)*u(2)*sqrt(u(1))
  Altitude effect on power : Fcn  Expr=u(3)*u(2)*sqrt(u(1))
  Constant10 : Constant  Value=mach_pow
  Constant4 : Constant  Value=mach_ffr
  Constant5 : Constant  Value=288.15
  Constant6 : Constant  Value=101325
  Constant7 : Constant  Value=elaw_2
  Constant8 : Constant  Value=elaw_1
  Constant9 : Constant  Value=elaw_0
  Divide : Product  Inputs=*/
  Divide1 : Product  Inputs=*/
  FFR law : Fcn  Expr=(u(2)*u(1)^2)+(u(3)*u(1))+u(4)
  Mach effect on FFR : Fcn  Expr=u(3)*(1+u(2)*u(1)^2)
  Mach effect on power : Fcn  Expr=u(3)*(1+u(2)*u(1)^2)
  Mux : Mux
  Mux{1..4} (4 alike) : Mux  Inputs=3
  Out1 : Outport
  Out2 : Outport  Port=2
  wires:
  Constant5/1 -> Divide/2
  Constant6/1 -> Divide1/2
  % throttle to FFR/1 -> Mux/1, Mux1/3
  Constant7/1 -> Mux/2
  Constant8/1 -> Mux/3
  Constant9/1 -> Mux/4
  Mux/1 -> FFR law/1
  Mux1/1 -> Mach effect on FFR/1
  Constant4/1 -> Mux1/2
  Mux2/1 -> Mach effect on power/1
  Constant10/1 -> Mux2/2
  FFR law/1 -> Mux2/3
  Divide/1 -> [theta]
  Divide1/1 -> [delta]
  [Mach] -> Mux1/1
  [Mach] -> Mux2/1
  Mux3/1 -> Altitude effect on FFR/1
  [theta] -> Mux3/1
  [delta] -> Mux3/2
  Mach effect on FFR/1 -> Mux3/3
  Mux4/1 -> Altitude effect on power/1
  [theta] -> Mux4/1
  [delta] -> Mux4/2
  Mach effect on power/1 -> Mux4/3
  In1/1 -> Divide1/1
  In2/1 -> [Mach]
  In3/1 -> Divide/1
  Altitude effect on FFR/1 -> Out1/1
  Altitude effect on power/1 -> Out2/1
  In4/1 -> % throttle to FFR/1
